simulink model "DiscreteController"  (R2021a)
settings: Solver=FixedStepAuto  StartTime=0.0  StopTime=600  FixedStep=1e-2  RelTol=1e-3
undefined symbols (not defined in the file or in its folder): Gc_Den, Gc_Num, Gd_Den_1, Gd_Den_2, Gd_Num_1, Gd_Num_2, Gp_Den, Gp_Num, Ts
settings Model: Creator=arman  LastModifiedBy=arman

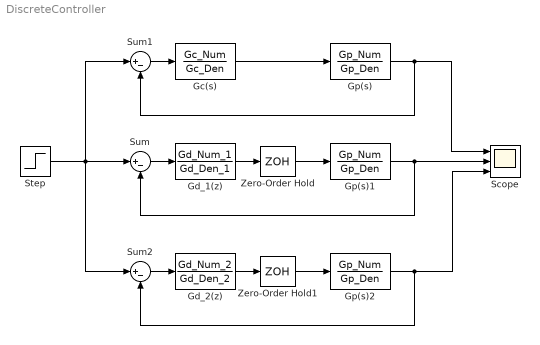
== system DiscreteController ==
  Gc(s) : TransferFcn  Numerator=Gc_Num  Denominator=Gc_Den
  Gd_1(z) : DiscreteTransferFcn  Numerator=Gd_Num_1  Denominator=Gd_Den_1  SampleTime=Ts
  Gd_2(z) : DiscreteTransferFcn  Numerator=Gd_Num_2  Denominator=Gd_Den_2  SampleTime=Ts
  Gp(s) : TransferFcn  Numerator=Gp_Num  Denominator=Gp_Den
  Gp(s)1 : TransferFcn  Numerator=Gp_Num  Denominator=Gp_Den
  Gp(s)2 : TransferFcn  Numerator=Gp_Num  Denominator=Gp_Den
  Scope : Scope  NumInputPorts=3
  Step : Step  SampleTime=0
  Sum : Sum  Inputs=|+-
  Sum1 : Sum  Inputs=|+-
  Sum2 : Sum  Inputs=|+-
  Zero-Order Hold : ZeroOrderHold  SampleTime=Ts
  Zero-Order Hold1 : ZeroOrderHold  SampleTime=Ts
  wires:
  Step/1 -> Sum2/1, Sum1/1, Sum/1
  Gc(s)/1 -> Gp(s)/1
  Sum1/1 -> Gc(s)/1
  Gp(s)/1 -> Sum1/2, Scope/1
  Zero-Order Hold/1 -> Gp(s)1/1
  Gp(s)1/1 -> Scope/2, Sum/2
  Gp(s)2/1 -> Scope/3, Sum2/2
  Zero-Order Hold1/1 -> Gp(s)2/1
  Sum/1 -> Gd_1(z)/1
  Gd_1(z)/1 -> Zero-Order Hold/1
  Sum2/1 -> Gd_2(z)/1
  Gd_2(z)/1 -> Zero-Order Hold1/1
